simulink model "new_pll_fs"  (Simulink 6.6)
settings: Solver=ode45  StartTime=0.0  StopTime=1.0  RelTol=1e-3
libraries: commsynccomp2 x1
settings Model: Creator=Administrator  LastModifiedBy=kostas777711

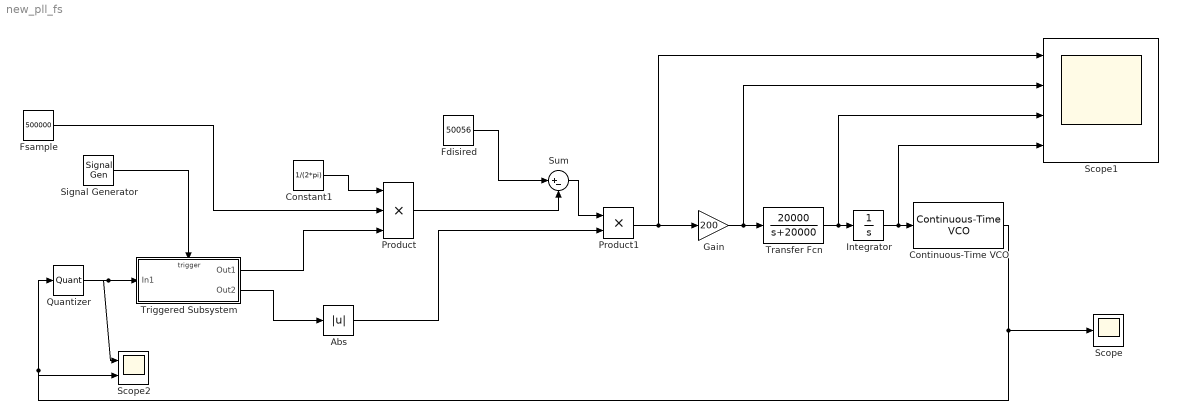
== system new_pll_fs ==
  Abs : Abs
  Constant1 : Constant  Value=1/(2*pi)
  Continuous-Time VCO : commsynccomp2/Continuous-Time VCO  SystemSampleTime=-1  Ac=1  Fc=10  Kc=1  Ph=0
  Fdisired : Constant  Value=50056
  Fsample : Constant  Value=500000
  Gain : Gain  Gain=200
  Integrator : Integrator
  Product : Product  Inputs=3  RndMeth=Zero
  Product1 : Product  RndMeth=Zero
  Quantizer : Quantizer  QuantizationInterval=2/(2^16)
  Scope : Scope
      settings: YMin=-2  YMax=2
  Scope1 : Scope  NumInputPorts=4
      settings: TimeRange=2e-006  YMin=87036.1~1.74072e+007~2.13871e+007~204414  YMax=87036.1~1.74072e+007~2.13871e+007~204414
  Scope2 : Scope  NumInputPorts=2
      settings: TimeRange=0.001  YMin=-1~-1  YMax=1~1  SaveName=ScopeData2
  Signal Generator : SignalGenerator  WaveForm=square  Frequency=500000
  Sum : Sum  Inputs=|+-
  Transfer Fcn : TransferFcn  Numerator=[20000]  Denominator=[1 20000]
  Triggered Subsystem : Subsystem  TreatAsAtomicUnit=on
  wires:
  Fsample/1 -> Product/2
  Constant1/1 -> Product/1
  Abs/1 -> Product1/2
  Product1/1 -> Gain/1, Scope1/1
  Fdisired/1 -> Sum/1
  Product/1 -> Sum/2
  Sum/1 -> Product1/1
  Gain/1 -> Transfer Fcn/1, Scope1/2
  Transfer Fcn/1 -> Integrator/1, Scope1/3
  Integrator/1 -> Continuous-Time VCO/1, Scope1/4
  Continuous-Time VCO/1 -> Scope/1, Quantizer/1, Scope2/2
  Signal Generator/1 -> Triggered Subsystem/Trigger
  Quantizer/1 -> Triggered Subsystem/1(In1), Scope2/1
  Triggered Subsystem/1(Out1) -> Product/3
  Triggered Subsystem/2(Out2) -> Abs/1

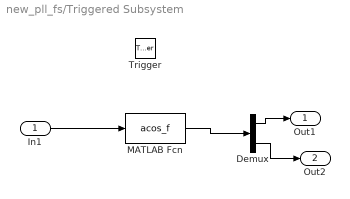
== system new_pll_fs/Triggered Subsystem ==
  In1 : Inport
  Trigger : TriggerPort
  Demux : Demux  Outputs=2
  MATLAB Fcn : MATLABFcn  MATLABFcn=acos_f
  Out1 : Outport
  Out2 : Outport  Port=2
  wires:
  In1/1 -> MATLAB Fcn/1
  MATLAB Fcn/1 -> Demux/1
  Demux/1 -> Out1/1
  Demux/2 -> Out2/1
